simulink model "Mooventure2016_Rev5"  (Simulink 7.7)
settings: Solver=FixedStepDiscrete  StartTime=0.0  StopTime=10  RelTol=1e-3
PreLoadFcn:
  | try, eval([bdroot '_setup']); catch, eval('model_setup', ''); end
InitFcn:
  | try, eval([bdroot '_setup']); catch, eval('model_setup', ''); end
undefined symbols (not defined in the file): ECM, H1, motohawk_build_version, motohawk_trunc_name, motohawk_vardec_config_group, motohawk_vardec_path, xD
libraries: MotoHawk_lib x976, motohawk_control_primitives_lib x41, simulink x27, motohawk_annotations_lib x3
(part 16 of 16)

== stateflow chart Foreground/Control/Coolant Control/BlendValving ==
  state SystemIdle
    during: RadiatorBlend=231;
    during: HeaterCoreBlend=20;
    during: Heat1=0;
    during: Heat2=0;
    during: Heat3=0;
    during: Heat4=0;
    during: RadiatorPump=0;
    during: HeaterCorePump=0;
  state SystemWarmup
    during: RadiatorBlend=231;
    during: HeaterCoreBlend=231;
    during: RadiatorPump=1;
    during: HeaterCorePump=1;
  state Heat1
    during: Heat1=1;
    during: Heat2=0;
    during: Heat3=0;
    during: Heat4=0;
  state Heat2
    during: Heat1=1;
    during: Heat2=1;
    during: Heat3=0;
    during: Heat4=0;
  state Heat4
    during: Heat1=1;
    during: Heat2=1;
    during: Heat3=1;
    during: Heat4=1;
  state Heat3
    during: Heat1=1;
    during: Heat2=1;
    during: Heat3=1;
    during: Heat4=0;
  state UserWantsHeat_NotHot
    during: HeaterCoreBlend=20;
    during: HeaterCorePump=1;
    during: Heat1=0;
    during: Heat2=0;
  state HeatOn
    during: Heat1=1;
    during: Heat2=1;
    during: Heat3=0;
    during: Heat4=0;
    during: HeaterCorePump=1;
    during: HeaterCoreBlend=20;
  (default) -> SystemIdle
  SystemIdle -> SystemWarmup [order 1] : [SystemCold==1]
  Heat1 -> SystemIdle [order 2] : [SystemWarm==1]
  SystemWarmup -> Heat1 [order 1] : [SystemCold==1 && (HeaterCorePump == 1) && (Heat1Threshold ~= 2000)]
  Heat1 -> Heat2 [order 1] : [HottestTemp<Heat2Threshold]
  Heat2 -> SystemIdle [order 3] : [SystemWarm==1]
  Heat3 -> Heat4 [order 1] : [HottestTemp<Heat4Threshold]
  Heat2 -> Heat3 [order 1] : [HottestTemp<Heat3Threshold]
  Heat4 -> Heat3 [order 1] : [HottestTemp>Heat4Threshold]
  Heat3 -> Heat2 [order 2] : [HottestTemp>Heat3Threshold]
  Heat2 -> Heat1 [order 2] : [HottestTemp>Heat2Threshold]
  SystemIdle -> UserWantsHeat_NotHot [order 2] : [!SystemCold && UserWantsHeat]
  UserWantsHeat_NotHot -> HeatOn [order 1] : [HeaterOutputTemp<(HeaterCoreThreshold+1)]
  HeatOn -> UserWantsHeat_NotHot [order 1] : [HeaterOutputTemp>(HeaterCoreThreshold-1)]
  UserWantsHeat_NotHot -> SystemIdle [order 2] : [!UserWantsHeat || (SystemCold && ~SomethingsHot)]
  HeatOn -> SystemIdle [order 2] : [UserWantsHeat==0 || SystemCold==1]
  Heat4 -> SystemIdle [order 2] : [SystemWarm==1]
  Heat3 -> SystemIdle [order 3] : [SystemWarm==1]
  SystemWarmup -> SystemIdle [order 2] : [SystemWarm==1]
  data: SystemCold input boolean; SystemWarm input boolean; RadiatorBlend output double; UserWantsHeat input boolean; HeaterCoreBlend output double; HeaterOutputTemp input double; HottestTemp input double; Heat1 output boolean; Heat2 output boolean; Heat3 output boolean; Heat4 output boolean; Heat1Threshold input double; Heat2Threshold input double; Heat3Threshold input double; Heat4Threshold input double; SomethingsHot input boolean; RadiatorPump output boolean; HeaterCorePump output boolean; HeaterCoreThreshold input double

== stateflow chart Foreground/Control/Hybrid Control Code/SUVMode/Chart ==
  state Nuetral
    during: driveTorque=0;
    during: regenTorque=0;
  state Driving
    during: driveTorque=accel;
    during: regenTorque=0;
  state RegenDrag
    during: regenTorque=dragTorque;
    during: driveTorque=0;
  state RegenBrake
    during: regenTorque=brake+dragTorque;
    during: driveTorque=0;
  (default) -> Nuetral
  Nuetral -> Driving : [accel>=accelStart]
  Driving -> RegenDrag : [accel<=accelEnd && speed>=regenStart]
  RegenDrag -> Nuetral [order 1] : [speed<=regenEnd]
  RegenBrake -> Nuetral [order 1] : [speed<=regenEnd]
  RegenDrag -> RegenBrake [order 2] : [brake>=brakeStart]
  RegenDrag -> Driving [order 3] : [accel>=accelStart]
  RegenBrake -> RegenDrag [order 2] : [brake<=brakeEnd]
  data: driveTorque output double; regenTorque output double; accel input double; brake input double; speed input double; accelStart input double; accelEnd input double; brakeStart input double; brakeEnd input double; regenStart input double; regenEnd input double; dragTorque input double

== matlab function Foreground/Inputs/Analog Inputs/Coolant/Embedded MATLAB Function ==
  data: thermistor_reading input double; temp_reading output double
function temp_reading = fcn(thermistor_reading)

temp_reading = 0.4254*thermistor_reading - 31.404;

== stateflow chart Foreground/Control/Coolant Control/PumpState ==
  state PumpOff
    during:
    PumpOn=false;
  state PumpOn
    during:
    PumpOn=true;
  (default) -> PumpOff
  PumpOff -> PumpOn : [SomethingsHot]
  PumpOn -> PumpOff : [SomethingsCold]
  data: SomethingsHot input boolean; SomethingsCold input boolean; PumpOn output boolean

== matlab function Foreground/Inputs/Driver Inputs/Embedded MATLAB Function ==
  data: posIn input double; posOut output double; ecoModeOut output double
function [posOut, ecoModeOut] = fcn(posIn)
% Park, Reverse, Drive, Low

if(posIn==12) 
    posOut=1;   % in reverse
    ecoModeOut=0;
elseif(posIn==8)
    posOut=3;   % in drive
    ecoModeOut=0;
elseif(posIn==4)
    posOut=3;   % in ecoMode drive
    ecoModeOut=1;
else
    posOut=2;   % in neutral
    ecoModeOut=0;
end

== matlab function Foreground/Control/Hybrid Control Code/SUVMode/Gas Pedal Scaling ==
  data: throttleIn input double; throttleOut output double
function throttleOut = fcn(throttleIn)
throttleOut=(throttleIn-16)/91;

== matlab function Foreground/Control/Hybrid Control Code/CrawlHomeMode/Brake Pedal Scaling ==
  data: brakeIn input double; brakeOut output double; inReverse input double
function brakeOut = fcn(brakeIn, inReverse)
if(~inReverse)
    brakeOut=1-((brakeIn-23900)/8900);
else
    brakeOut=1-((41700-brakeIn)/8900);
end

== matlab function Foreground/Control/Hybrid Control Code/EcoMode/Brake Pedal Scaling ==
  data: brakeIn input double; brakeOut output double; inReverse input double
function brakeOut = fcn(brakeIn, inReverse)
if(~inReverse)
    brakeOut=1-((brakeIn-23900)/8900);
else
    brakeOut=1-((41700-brakeIn)/8900);
end

== stateflow chart Foreground/Control/Hybrid Control Code/CrawlHomeMode/Chart ==
  state Nuetral
    during: driveTorque=0;
    during: regenTorque=0;
  state Driving
    during: driveTorque=accel;
    during: regenTorque=0;
  state RegenDrag
    during: regenTorque=dragTorque;
    during: driveTorque=0;
  state RegenBrake
    during: regenTorque=brake+dragTorque;
    during: driveTorque=0;
  (default) -> Nuetral
  Nuetral -> Driving : [accel>=accelStart]
  Driving -> RegenDrag : [accel<=accelEnd && speed>=regenStart]
  RegenDrag -> Nuetral [order 1] : [speed<=regenEnd]
  RegenBrake -> Nuetral [order 1] : [speed<=regenEnd]
  RegenDrag -> RegenBrake [order 2] : [brake>=brakeStart]
  RegenDrag -> Driving [order 3] : [accel>=accelStart]
  RegenBrake -> RegenDrag [order 2] : [brake<=brakeEnd]
  data: driveTorque output double; regenTorque output double; accel input double; brake input double; speed input double; accelStart input double; accelEnd input double; brakeStart input double; brakeEnd input double; regenStart input double; regenEnd input double; dragTorque input double

== matlab function Foreground/Control/Hybrid Control Code/CrawlHomeMode/Gas Pedal Scaling ==
  data: throttleIn input double; throttleOut output double
function throttleOut = fcn(throttleIn)
throttleOut=(throttleIn-16)/91;

== stateflow chart Foreground/Outputs/Driver Ouputs/Chart ==
  state Normal
    during: engTemp=23;
    during: transTemp=23;
  state Solid
    during: engTemp=200;
    during: transTemp=200;
  state FlashOn
    during: engTemp=200;
    during: transTemp=200;
  state FlashOff
    during: engTemp=23;
    during: transTemp=23;
    during: timerOut=0;
  state Wait
    during: timerOut=1;
  (default) -> Normal
  Normal -> Solid [order 1] : [solid==1]
  Solid -> Normal : [solid==0]
  Normal -> FlashOn [order 2] : [flash==1]
  FlashOn -> Normal [order 1] : [flash==0]
  FlashOff -> Normal : [flash==0]
  FlashOn -> Wait [order 2] : [engTemp==200]
  Wait -> FlashOff : [timerIn==1]
  data: engTemp output double; transTemp output double; solid input double; flash input double; timerIn input boolean; timerOut output double

== matlab function Foreground/Outputs/Coolant Outputs/Radiator Motion Control ==
  data: currPos input double; motorEnable output double; posRequest input double; motorDirection output double; hyst input double
function [motorEnable, motorDirection] = fcn(currPos, posRequest, hyst)

if(currPos<=posRequest+hyst && currPos>=posRequest-hyst)
    motorEnable=0;
    motorDirection=0;
elseif(currPos<posRequest)
    motorEnable=1;
    motorDirection=0;
elseif(currPos>posRequest)
    motorEnable=1;
    motorDirection=1;
else
    motorEnable=0;
    motorDirection=0;
end

== matlab function Foreground/Outputs/Coolant Outputs/Heater Core Motion Control ==
  data: currPos input double; motorEnable output double; posRequest input double; motorDirection output double; hyst input double
function [motorEnable, motorDirection] = fcn(currPos, posRequest, hyst)

if(currPos<=posRequest+hyst && currPos>=posRequest-hyst)
    motorEnable=0;
    motorDirection=0;
elseif(currPos<posRequest)
    motorEnable=1;
    motorDirection=0;
elseif(currPos>posRequest)
    motorEnable=1;
    motorDirection=1;
else
    motorEnable=0;
    motorDirection=0;
end

== matlab function Foreground/Control/Hybrid Control Code/Embedded MATLAB Function ==
  data: set_crawl_home input double; current_state input double; state output double
function state = fcn(set_crawl_home, current_state)
    if(set_crawl_home)
        state = 1;
    else
        state = current_state;
    end

== matlab function Foreground/Control/Coolant Control/Embedded MATLAB Function ==
  data: sHot input double; radBlend output double; pass input double
function radBlend = fcn(sHot,pass)

if(sHot)
    radBlend=20;
elseif(pass>=30)
    radBlend=pass;
else
    radBlend=231;
end

== matlab function Foreground/Control/Coolant Control/Embedded MATLAB Function1 ==
  data: maxTemp input double; radiatorFan output double; lowThreshold input double; mediumThreshold input double; highThreshold input double; acOn input double; fault input double; engineTemp input double
function radiatorFan = fcn(maxTemp, lowThreshold, mediumThreshold, highThreshold, acOn, fault, engineTemp)

if(fault==1 || acOn==1)
    radiatorFan=3;
elseif(maxTemp<lowThreshold || engineTemp<lowThreshold)
    radiatorFan=0;
elseif((maxTemp>=lowThreshold && maxTemp<mediumThreshold) || (engineTemp>=lowThreshold+25 && engineTemp<mediumThreshold+25))
    radiatorFan=1;
elseif((maxTemp>=mediumThreshold && maxTemp<highThreshold) || (engineTemp>=mediumThreshold+25 && engineTemp<highThreshold+25))
    radiatorFan=2;
elseif((maxTemp>=highThreshold) || engineTemp>=highThreshold+25)
    radiatorFan=3;
else
    radiatorFan=0;
end

== stateflow chart Foreground/Outputs/Driver Ouputs/PowerSteering ==
  state INIT
    during:
    VehicleReadyOutput=false;
  state MotorRunning
    during:
    VehicleReadyOutput=true;
  state PowerSteeringOn
    during:
    VehicleReadyOutput=true;
  state PowerSteeringOff
    during:
    VehicleReadyOutput=false;
  (default) -> INIT
  INIT -> MotorRunning : [MotorReady]
  MotorRunning -> PowerSteeringOn : [~VehicleReadyInput]
  PowerSteeringOn -> PowerSteeringOff : [ShiftPosition==2]
  data: VehicleReadyInput input boolean; ShiftPosition input double; MotorReady input boolean; VehicleReadyOutput output boolean

== stateflow chart Foreground/Inputs/Cruise Control/Chart ==
  state default
    during: Out=0;
  state Off
    during: Out=1;
  state SetMinus
    during: Out=2;
  state SetPlus
    during: Out=3;
  state RSM
    during: Out=4;
  state ON
    during: Out=5;
  (default) -> default
  default -> Off [order 1] : [Switch<Off+HYST && Switch>Off-HYST]
  ON -> default : [Switch<Default+HYST && Switch>Default-HYST]
  SetMinus -> default : [Switch<Default+HYST && Switch>Default-HYST]
  default -> SetMinus [order 5] : [Switch<SetMinus+HYST && Switch>SetMinus-HYST]
  default -> SetPlus [order 2] : [Switch<SetPlus+HYST && Switch>SetPlus-HYST]
  SetPlus -> default : [Switch<Default+HYST && Switch>Default-HYST]
  default -> RSM [order 3] : [Switch<RSM+HYST && Switch>RSM-HYST]
  RSM -> default : [Switch<Default+HYST && Switch>Default-HYST]
  default -> ON [order 4] : [Switch<ON+HYST && Switch>ON-HYST]
  Off -> default : [Switch<Default+HYST && Switch>Default-HYST]
  data: Switch input double; Off input double; SetMinus input double; SetPlus input double; RSM input double; ON input double; HYST input double; Out output double; Default input double

== stateflow chart Foreground/Control/Hybrid Control Code/Cruise Control/SystemState ==
  state Off
    during: System=0;
  state On
    during: System=1;
  (default) -> Off
  Off -> On : [CruiseOn==1 && CruiseEnable==1]
  On -> Off : [CruiseOff==1 || CruiseEnable==0]
  data: CruiseOff input boolean; System output boolean; CruiseOn input boolean; CruiseEnable input boolean

== matlab function Foreground/Control/Hybrid Control Code/Traction Control/Torque Limiter ==
  data: maxTorque input double; torqueIn input double; torqueOut output double
function torqueOut = fcn(maxTorque, torqueIn)

if abs(torqueIn) <  maxTorque
    torqueOut = torqueIn;
elseif abs(torqueIn) >= maxTorque
    torqueOut = maxTorque*sign(torqueIn);
else
    torqueOut = torqueIn;
end

== matlab function Foreground/Outputs/ABS Outputs/Shift Position Conditioner ==
  data: dirOut output double; dirIn input double
function dirOut = fcn(dirIn)

if dirIn == 1
    dirOut = 0;
else
    dirOut = 1;
end

== stateflow chart Foreground/Control/Engine Control/Chart ==
  state default
    du: Genset_Enable = 0;
    Genset_Load = 0;
    Genset_RPM = 0;
    Genset_Throttle = 0;
  state Startup
    du: Genset_Enable = 1;
  state Running
    du: Genset_Load = 1;
    state default_gen
      du: Genset_RPM = 0;
      Genset_Throttle = 0;
    state low_gen
      du: Genset_RPM = Low_RPM;
      Genset_Throttle = Low_Throttle;
    state medium_gen
      du: Genset_RPM = Medium_RPM;
      Genset_Throttle = Medium_Throttle;
    state high_gen
      du: Genset_RPM = High_RPM;
      Genset_Throttle = High_Throttle;
    (default) -> default_gen
    default_gen -> low_gen : [Coolant_Temp > Coolant_Cold]
    low_gen -> medium_gen [order 1] : [Coolant_Temp > Coolant_Warm]
    medium_gen -> high_gen [order 1] : [(Coolant_Temp > Coolant_Hot) && SOC_Critical]
    high_gen -> medium_gen [order 1] : [!SOC_Critical]
    medium_gen -> low_gen [order 2] : [Coolant_Temp < (Coolant_Warm-3)]
    low_gen -> default_gen [order 2] : [(Coolant_Temp < (Coolant_Cold -3)) || SOC_High || Speed_Off]
    medium_gen -> default_gen [order 3] : [SOC_High || Speed_Off]
    high_gen -> default_gen [order 2] : [SOC_High]
  state Shutdown
    du: Genset_Enable = 0;
    Genset_Throttle = 0;
    Genset_RPM = 0;
  (default) -> default
  default -> Startup : [SOC_Critical || (SOC_Low && Speed_On)]
  Startup -> Running : [Engine_On]
  Running -> Shutdown : [SOC_High || (Speed_Off && !SOC_Critical)]
  Shutdown -> default : [Engine_RPM < 200]
  data: SOC_Low input double; SOC_High input double; SOC_Critical input double; Speed_On input double; Speed_Off input double; SOC input double; Coolant_Temp input double; Coolant_Cold input double; Coolant_Warm input double; Coolant_Hot input double; Low_RPM input double; Medium_RPM input double; High_RPM input double; Low_Throttle input double; Medium_Throttle input double; High_Throttle input double; Genset_Enable output double; Genset_Load output double; Genset_RPM output double; Genset_Throttle output double; Engine_On input double; Engine_RPM input double

== matlab function Foreground/Control/Faults/Power Train/Vehicle Speed Sensor/Data Correction ==
  data: torqueIn input double; torqueOut output double
function torqueOut = fcn(torqueIn)

if torqueIn > 0
    torqueOut = -(4000-torqueIn);
elseif torqueIn < 0
    torqueOut = -(-4000-torqueIn);
else
    torqueOut = 0;
end

== matlab function Foreground/Outputs/Driver Ouputs/Embedded MATLAB Function ==
  data: solid input double; CEL output double; flashing input double
function CEL = fcn(solid,flashing)

if flashing == 1
    CEL = 2;
elseif solid == 1
    CEL = 1;
else
    CEL = 0;
end

== stateflow chart Foreground/Outputs/Driver Ouputs/Enabled Subsystem/Bar Chart Reset ==
  state Init
    during: write=0;
  state Counting
    during: count++;
  state Write
    during: write=1;
  state Clear
    during: write=0;
    during: count=0;
  (default) -> Init
  Init -> Counting : [write==0]
  Counting -> Write : [count>=delay]
  Write -> Clear : [write==1]
  Clear -> Init : [write==0]
  data: write output boolean; count local double; delay input double

== matlab function Foreground/Control/Faults/Freeze Frame/Data Write/Data Iterator ==
  data: dataIn input double; data output double; row output double; col output double; currentRow input double
function [data,row,col] = fcn(dataIn,currentRow)

row = currentRow+1;
for i = 1:6
    col = i;
    data = dataIn(i);
end

== matlab function Foreground/Control/Faults/Power Train/Electric Motor/Data Correction Motor Fault ==
  data: torqueIn input double; torqueOut output double
function torqueOut = fcn(torqueIn)

if torqueIn > 0
    torqueOut = -(4000-torqueIn);
elseif torqueIn < 0
    torqueOut = -(-4000-torqueIn);
else
    torqueOut = 0;
end

== matlab function Foreground/Outputs/Coolant Outputs/Fan Adapter ==
  data: speed input double; fan1 output double; fan2 output double; fan3 output double
function [fan1,fan2,fan3] = fcn(speed)

if speed == 1
    fan1 = 1;
    fan2 = 0;
    fan3 = 0;
elseif speed == 2
    fan1 = 0;
    fan2 = 1;
    fan3 = 0;
elseif speed == 3
    fan1 = 0;
    fan2 = 1;
    fan3 = 1;
else
    fan1 = 0;
    fan2 = 0;
    fan3 = 0;
end

== matlab function Foreground/Outputs/ABS Outputs/Data Correction Motor ABS ==
  data: torqueIn input double; torqueOut output double
function torqueOut = fcn(torqueIn)

if torqueIn > 0
    torqueOut = -(4000-torqueIn);
elseif torqueIn < 0
    torqueOut = -(-4000-torqueIn);
else
    torqueOut = 0;
end

== matlab function Foreground/Outputs/Driver Ouputs/ODO_CALC ==
  data: dist input double; reset output double; ODO_in input double; ODO_out output double
function [reset,ODO_out] = fcn(dist,ODO_in)

if dist >= 0.016666666
    if ODO_in - 0.0001 <= 0
        ODO_out = (0.05 + ODO_in) - 0.0001;
        reset = 0 ;
    else
        ODO_out = ODO_in - 0.0001;
        reset = 0 ;
    end
else
    ODO_out = ODO_in;
    reset = dist;
end
